simulink model "sim_RLC"  (R2022a)
settings: Solver=VariableStepAuto  StartTime=0.0  StopTime=0.5  MaxStep=1e-4  RelTol=1e-3
undefined symbols (not defined in the file or in its folder): A, B, den, den1, den2, num, num1, num2
settings Model: Creator=PSCAD_FAN  LastModifiedBy=PSCAD_FAN

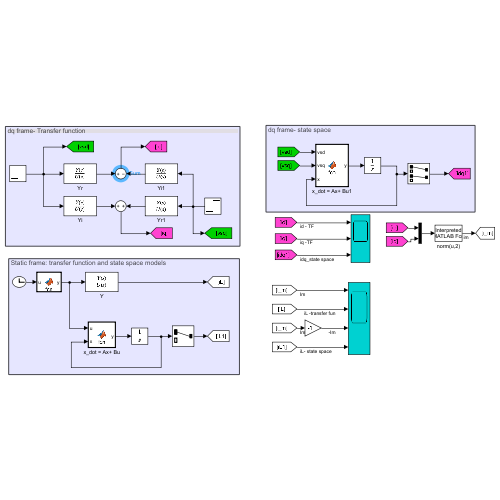
[thumbnail: Simulink's stored preview of the top-level diagram]
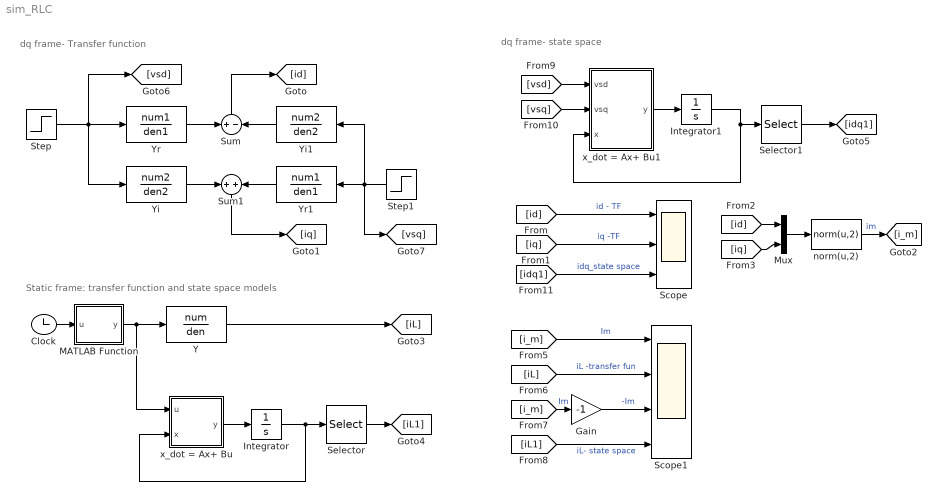
== system sim_RLC ==
  note: Static frame: transfer function and state space models
  note: dq frame- state space
  note: dq frame- Transfer function
  Clock : Clock
  Gain : Gain  Gain=-1
  Integrator : Integrator
  Integrator1 : Integrator
  MATLAB Function : MATLAB Function  TreatAsAtomicUnit=on
  Mux : Mux  Inputs=2
  Scope : Scope  NumInputPorts=3
  Scope1 : Scope  NumInputPorts=4
  Selector : Selector  InputPortWidth=2  IndexOptions=Index vector (dialog)  Indices=[1]  OutputSizes=1
  Selector1 : Selector  InputPortWidth=4  IndexOptions=Index vector (dialog)  Indices=[1 3]  OutputSizes=1
  Step : Step  Time=0.1  SampleTime=0
  Step1 : Step  After=0  SampleTime=0
  Sum : Sum  Inputs=+-
  Sum1 : Sum
  Y : TransferFcn  Numerator=num  Denominator=den
  Yi : TransferFcn  Numerator=num2  Denominator=den2
  Yi1 : TransferFcn  Numerator=num2  Denominator=den2
  Yr : TransferFcn  Numerator=num1  Denominator=den1
  Yr1 : TransferFcn  Numerator=num1  Denominator=den1
  norm(u,2) : MATLABFcn  MATLABFcn=norm(u,2)
  x_dot = Ax+ Bu : MATLAB Function  TreatAsAtomicUnit=on
  x_dot = Ax+ Bu1 : MATLAB Function  TreatAsAtomicUnit=on
  wires:
  Step/1 -> [vsd], Yi/1, Yr/1
  Step1/1 -> [vsq], Yr1/1, Yi1/1
  Yr/1 -> Sum/1
  Yi1/1 -> Sum/2
  Yr1/1 -> Sum1/2
  Yi/1 -> Sum1/1
  Sum1/1 -> [iq]
  Sum/1 -> [id]
  Mux/1 -> norm(u,2)/1
  [id] -> Mux/1
  [iq] -> Mux/2
  norm(u,2)/1 -> [i_m]  "im"
  Y/1 -> [iL]
  Clock/1 -> MATLAB Function/1(u)
  MATLAB Function/1(y) -> x_dot = Ax+ Bu/1(u), Y/1
  [i_m] -> Scope1/1  "Im"
  [iL] -> Scope1/2  "iL -transfer fun"
  Gain/1 -> Scope1/3  "-Im"
  [i_m] -> Gain/1  "Im"
  x_dot = Ax+ Bu/1(y) -> Integrator/1
  Integrator/1 -> Selector/1, x_dot = Ax+ Bu/2(x)
  Selector/1 -> [iL1]
  [iL1] -> Scope1/4  "iL- state space"
  Selector1/1 -> [idq1]
  Integrator1/1 -> Selector1/1, x_dot = Ax+ Bu1/3(x)
  x_dot = Ax+ Bu1/1(y) -> Integrator1/1
  [vsd] -> x_dot = Ax+ Bu1/1(vsd)
  [vsq] -> x_dot = Ax+ Bu1/2(vsq)
  [id] -> Scope/1  "id - TF"
  [iq] -> Scope/2  "iq -TF"
  [idq1] -> Scope/3  "idq_state space"

== matlab function sim_RLC/x_dot = Ax+ Bu ==
  data: u input; y output; x input; A parameter; B parameter
function y = fcn(u, x, A, B)

y = A*x+B*u;

== matlab function sim_RLC/MATLAB Function ==
  data: u input; y output
function y = fcn(u)
if (u<0.1)
    y=0;
else
y = cos(377*u);
end

== matlab function sim_RLC/x_dot = Ax+ Bu1 ==
  data: vsd input; vsq input; y output; x input; A parameter; B parameter
function y = fcn(vsd, vsq, x, A, B)

n = length(x)/2; 
x1= x(1:n)+1i*x(n+1:2*n);
u = vsd+1i*vsq; 
temp = (A- 1i*377*eye(2))*x1+B*u;
y = [real(temp); imag(temp)];
